simulink model "week2_1"  (R2020b)
settings: Solver=VariableStepAuto  StartTime=0.0  StopTime=10.0  RelTol=1e-3
settings Model: Creator=MY lenovo  LastModifiedBy=MY lenovo

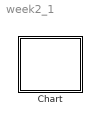
== system week2_1 ==
  Chart : Stateflow chart  TreatAsAtomicUnit=on

== stateflow chart week2_1/Chart ==
  state state1
    en:o1=0;
    o2=0;
    o3=0;
  (default) -> state1
